simulink model "project"  (R2021a)
settings: Solver=VariableStepAuto  StartTime=0.0  StopTime=10.0  RelTol=1e-3
libraries: custom_lib x17
settings Model: Creator=Acer  LastModifiedBy=Acer

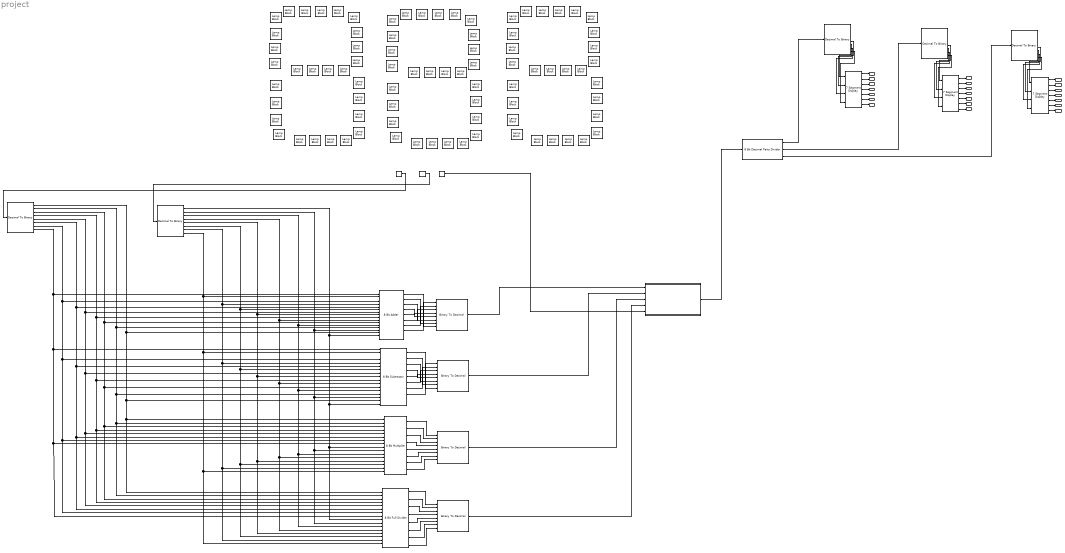
== system project ==
  7 Segment Display : custom_lib/7 Segment Display  SystemSampleTime=-1  VariantActivationTime=update diagram  Latency=0  AutoFrameSizeCalculation=off
      settings: SourceProductName=Custom Library
  7 Segment Display1 : custom_lib/7 Segment Display  SystemSampleTime=-1  VariantActivationTime=update diagram  Latency=0  AutoFrameSizeCalculation=off
      settings: SourceProductName=Custom Library
  7 Segment Display2 : custom_lib/7 Segment Display  SystemSampleTime=-1  VariantActivationTime=update diagram  Latency=0  AutoFrameSizeCalculation=off
      settings: SourceProductName=Custom Library
  8 Bit Adder : custom_lib/8 Bit Adder  SystemSampleTime=-1  VariantActivationTime=update diagram  Latency=0  AutoFrameSizeCalculation=off
      settings: SourceProductName=Custom Library
  8 Bit Decimal Parts Divider : custom_lib/8 Bit Decimal Parts Divider  SystemSampleTime=-1  VariantActivationTime=update diagram  Latency=0  AutoFrameSizeCalculation=off
      settings: SourceProductName=Custom Library
  8 Bit Full Divider : custom_lib/8 Bit Full Divider  SystemSampleTime=-1  VariantActivationTime=update diagram  Latency=0  AutoFrameSizeCalculation=off
      settings: SourceProductName=Custom Library
  8 Bit Multiplier : custom_lib/8 Bit Multiplier  SystemSampleTime=-1  VariantActivationTime=update diagram  Latency=0  AutoFrameSizeCalculation=off
      settings: SourceProductName=Custom Library
  8 Bit Subtractor : custom_lib/8 Bit Subtractor  SystemSampleTime=-1  VariantActivationTime=update diagram  Latency=0  AutoFrameSizeCalculation=off
      settings: SourceProductName=Custom Library
  A : Constant  Value=88
  B : Constant  Value=3
  Binary To Decimal{,1..3} (4 alike) : custom_lib/Binary To Decimal  SystemSampleTime=-1  VariantActivationTime=update diagram  Latency=0  AutoFrameSizeCalculation=off
      settings: SourceProductName=Custom Library
  Decimal To Binary{,1,4..6} (5 alike) : custom_lib/Decimal To Binary  SystemSampleTime=-1  VariantActivationTime=update diagram  Latency=0  AutoFrameSizeCalculation=off
      settings: SourceProductName=Custom Library
  Lamp{,1..83} (84 alike) : LampBlock
  Operation : Constant  Value=4
  Operation Decider : MATLAB Function  TreatAsAtomicUnit=on
  Output : Outport
  Output1 : Outport  Port=2
  Output2 : Outport  Port=3
  Output3 : Outport  Port=4
  Output4 : Outport  Port=5
  Output5 : Outport  Port=6
  Output6 : Outport  Port=7
  Output7 : Outport  Port=8
  Output8 : Outport  Port=9
  Output9 : Outport  Port=10
  Output10 : Outport  Port=11
  Output11 : Outport  Port=12
  Output12 : Outport  Port=13
  Output13 : Outport  Port=14
  Output14 : Outport  Port=15
  Output15 : Outport  Port=16
  Output16 : Outport  Port=17
  Output17 : Outport  Port=18
  Output18 : Outport  Port=19
  Output19 : Outport  Port=20
  Output20 : Outport  Port=21
  wires:
  8 Bit Adder/1 -> Binary To Decimal/8
  8 Bit Adder/2 -> Binary To Decimal/7
  8 Bit Adder/3 -> Binary To Decimal/6
  8 Bit Adder/4 -> Binary To Decimal/5
  8 Bit Adder/5 -> Binary To Decimal/4
  8 Bit Adder/6 -> Binary To Decimal/3
  8 Bit Adder/7 -> Binary To Decimal/2
  8 Bit Adder/8 -> Binary To Decimal/1
  8 Bit Subtractor/7 -> Binary To Decimal1/2
  8 Bit Subtractor/3 -> Binary To Decimal1/6
  8 Bit Subtractor/6 -> Binary To Decimal1/3
  8 Bit Subtractor/4 -> Binary To Decimal1/5
  8 Bit Subtractor/8 -> Binary To Decimal1/1
  8 Bit Subtractor/2 -> Binary To Decimal1/7
  8 Bit Subtractor/1 -> Binary To Decimal1/8
  8 Bit Subtractor/5 -> Binary To Decimal1/4
  7 Segment Display/1 -> Output/1
  7 Segment Display/2 -> Output1/1
  7 Segment Display/3 -> Output2/1
  7 Segment Display/4 -> Output3/1
  7 Segment Display/5 -> Output4/1
  7 Segment Display/6 -> Output5/1
  7 Segment Display/7 -> Output6/1
  Decimal To Binary4/8 -> 7 Segment Display/4
  Decimal To Binary4/7 -> 7 Segment Display/3
  Decimal To Binary4/6 -> 7 Segment Display/2
  Decimal To Binary4/5 -> 7 Segment Display/1
  7 Segment Display1/4 -> Output10/1
  7 Segment Display1/1 -> Output7/1
  Decimal To Binary5/7 -> 7 Segment Display1/3
  Decimal To Binary5/6 -> 7 Segment Display1/2
  7 Segment Display1/7 -> Output13/1
  7 Segment Display1/5 -> Output11/1
  7 Segment Display1/6 -> Output12/1
  Decimal To Binary5/8 -> 7 Segment Display1/4
  Decimal To Binary5/5 -> 7 Segment Display1/1
  7 Segment Display1/3 -> Output9/1
  7 Segment Display1/2 -> Output8/1
  7 Segment Display2/6 -> Output19/1
  Decimal To Binary6/5 -> 7 Segment Display2/1
  Decimal To Binary6/8 -> 7 Segment Display2/4
  Decimal To Binary6/6 -> 7 Segment Display2/2
  7 Segment Display2/1 -> Output14/1
  7 Segment Display2/7 -> Output20/1
  7 Segment Display2/5 -> Output18/1
  7 Segment Display2/3 -> Output16/1
  Decimal To Binary6/7 -> 7 Segment Display2/3
  7 Segment Display2/2 -> Output15/1
  7 Segment Display2/4 -> Output17/1
  8 Bit Decimal Parts Divider/1 -> Decimal To Binary4/1
  8 Bit Decimal Parts Divider/2 -> Decimal To Binary5/1
  8 Bit Decimal Parts Divider/3 -> Decimal To Binary6/1
  Decimal To Binary/8 -> 8 Bit Adder/1, 8 Bit Subtractor/1, 8 Bit Full Divider/8, 8 Bit Multiplier/8
  Decimal To Binary/7 -> 8 Bit Adder/4, 8 Bit Full Divider/7, 8 Bit Multiplier/7, 8 Bit Subtractor/4
  Decimal To Binary/5 -> 8 Bit Full Divider/5, 8 Bit Multiplier/5, 8 Bit Subtractor/8, 8 Bit Adder/8
  Decimal To Binary/6 -> 8 Bit Adder/6, 8 Bit Full Divider/6, 8 Bit Multiplier/6, 8 Bit Subtractor/6
  Decimal To Binary/4 -> 8 Bit Full Divider/4, 8 Bit Multiplier/4, 8 Bit Subtractor/10, 8 Bit Adder/10
  Decimal To Binary/3 -> 8 Bit Full Divider/3, 8 Bit Multiplier/3, 8 Bit Subtractor/12, 8 Bit Adder/12
  Decimal To Binary/2 -> 8 Bit Full Divider/2, 8 Bit Multiplier/2, 8 Bit Subtractor/14, 8 Bit Adder/14
  Decimal To Binary/1 -> 8 Bit Full Divider/1, 8 Bit Multiplier/1, 8 Bit Subtractor/16, 8 Bit Adder/16
  Decimal To Binary1/8 -> 8 Bit Full Divider/16, 8 Bit Multiplier/16, 8 Bit Subtractor/2, 8 Bit Adder/2
  Decimal To Binary1/7 -> 8 Bit Adder/5, 8 Bit Full Divider/15, 8 Bit Multiplier/15, 8 Bit Subtractor/5
  Decimal To Binary1/6 -> 8 Bit Adder/7, 8 Bit Full Divider/14, 8 Bit Multiplier/14, 8 Bit Subtractor/7
  Decimal To Binary1/5 -> 8 Bit Adder/9, 8 Bit Full Divider/13, 8 Bit Multiplier/13, 8 Bit Subtractor/9
  Decimal To Binary1/4 -> 8 Bit Adder/11, 8 Bit Full Divider/12, 8 Bit Multiplier/12, 8 Bit Subtractor/11
  Decimal To Binary1/3 -> 8 Bit Adder/13, 8 Bit Full Divider/11, 8 Bit Multiplier/11, 8 Bit Subtractor/13
  Decimal To Binary1/2 -> 8 Bit Adder/15, 8 Bit Full Divider/10, 8 Bit Multiplier/10, 8 Bit Subtractor/15
  Decimal To Binary1/1 -> 8 Bit Full Divider/9, 8 Bit Multiplier/9, 8 Bit Subtractor/17, 8 Bit Adder/17
  A/1 -> Decimal To Binary/1
  B/1 -> Decimal To Binary1/1
  8 Bit Multiplier/8 -> Binary To Decimal2/8
  8 Bit Multiplier/7 -> Binary To Decimal2/7
  8 Bit Multiplier/6 -> Binary To Decimal2/6
  8 Bit Multiplier/5 -> Binary To Decimal2/5
  8 Bit Multiplier/4 -> Binary To Decimal2/4
  8 Bit Multiplier/3 -> Binary To Decimal2/3
  8 Bit Multiplier/2 -> Binary To Decimal2/2
  8 Bit Multiplier/1 -> Binary To Decimal2/1
  8 Bit Full Divider/8 -> Binary To Decimal3/8
  8 Bit Full Divider/7 -> Binary To Decimal3/7
  8 Bit Full Divider/6 -> Binary To Decimal3/6
  8 Bit Full Divider/5 -> Binary To Decimal3/5
  8 Bit Full Divider/4 -> Binary To Decimal3/4
  8 Bit Full Divider/3 -> Binary To Decimal3/3
  8 Bit Full Divider/2 -> Binary To Decimal3/2
  8 Bit Full Divider/1 -> Binary To Decimal3/1
  Operation Decider/1(out) -> 8 Bit Decimal Parts Divider/1
  Operation/1 -> Operation Decider/5(operation)
  Binary To Decimal/1 -> Operation Decider/1(sum)
  Binary To Decimal1/1 -> Operation Decider/2(diff)
  Binary To Decimal2/1 -> Operation Decider/3(prod)
  Binary To Decimal3/1 -> Operation Decider/4(quo)

== matlab function project/Operation Decider ==
  data: sum input; diff input; prod input; quo input; out output; operation input
function out  = fcn(sum, diff, prod, quo, operation)

switch operation
    case 1
        out = sum;
    case 2
        out = diff;
    case 3
        out = prod;
    otherwise
        out = quo;
end
